simulink model "Model2_V032_R_T4"  (R2023a)
settings: Solver=ode14x  StartTime=0.0  StopTime=Inf  FixedStep=ts  MaxStep=ts  RelTol=1e-5
values from neighbouring files (symbols this model uses):
  ausrollen_a_v = parameters.ausrollen_a_v    [efficiencycalc.m]    (also in parameters_initials.mat = 1)
  bremspunkte = parameters.bremspunkte    [efficiencycalc.m]    (also in parameters_initials.mat = [6100  280  8; 10400  500  3; 14100  550  8; 17729  0  1])
  brennstoffzellen_eta_kennfeld = parameters.brennstoffzellen_eta_kennfeld    [efficiencycalc.m]    (also in parameters_initials.mat = )
  brennstoffzellen_ui_kennfeld = parameters.brennstoffzellen_ui_kennfeld    [efficiencycalc.m]    (also in parameters_initials.mat = )
  coeffs_motor_moment = parameters.coeffs_motor_moment    [efficiencycalc.m]    (also in parameters_initials.mat = [30 30 30 5 7.5 10 0 0 0 6000 6000 6000 ... (30 elements, 3x)
  coeffs_motor_wirkungsgrad = parameters.coeffs_motor_wirkungsgrad    [efficiencycalc.m]    (also in parameters_initials.mat = [30 30 30 5 7.5 10 0 0 0 6000 6000 6000 ... (39 elements, 3x)
  fahrzeug_parameter = parameters.fahrzeug_parameter    [efficiencycalc.m]    (also in parameters_initials.mat = )
  strategie_parameter = parameters.strategie_parameter    [efficiencycalc.m]    (also in parameters_initials.mat = )
  strecke = parameters.strecke    [efficiencycalc.m]    (also in parameters_initials.mat = )
  ts = parameters.ts    [efficiencycalc.m]    (also in parameters_initials.mat = 0.01)
  U_moment = parameters.U_moment    [efficiencycalc.m]    (also in parameters_initials.mat = [30 3])
  U_wirkungsgrad = parameters.U_wirkungsgrad    [efficiencycalc.m]    (also in parameters_initials.mat = [30 3])
  umwelt_parameter = parameters.umwelt_parameter    [efficiencycalc.m]    (also in parameters_initials.mat = )
  zwangsgas = zeros(length(strecke.x),strecke.Rundenzahl)    [Automatisierung_Model_2.m]    (also in efficiencycalc.m; parameters_initials.mat = [0 0 0 0 0 0 0 0 0 0 0 0 ... (2563 elements, 233x11)])
libraries: simulink x1
(part 1 of 3)
settings Model: Creator=Robin Nedella  LastModifiedBy=Fer
settings SolverCC: NumberNewtonIterations=5  AlgebraicLoopSolver=LineSearch
settings DataIOCC: ReturnWorkspaceOutputs=off
settings DebuggingCC: ParameterOverflowMsg=none  UnderSpecifiedDimensionMsg=warning  ArithmeticOperatorsInVariantConditions=warning
settings ModelReferenceCC: EnableRefExpFcnMdlSchedulingChecks=on
settings SFSimCC: SimUseLocalCustomCode=off  CustomCodeUndefinedFunction=UseInterfaceOnly
settings RTWCC: RTWUseLocalCustomCode=off

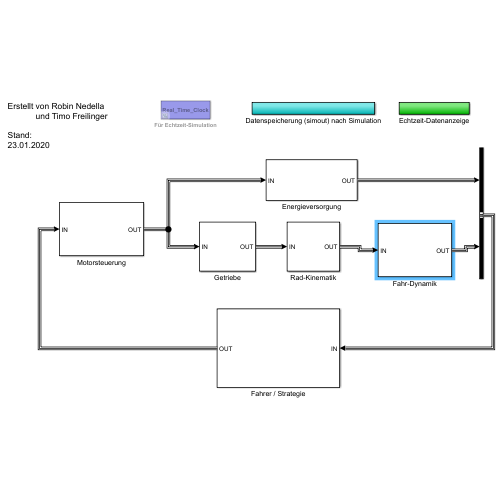
[thumbnail: Simulink's stored preview of the top-level diagram]
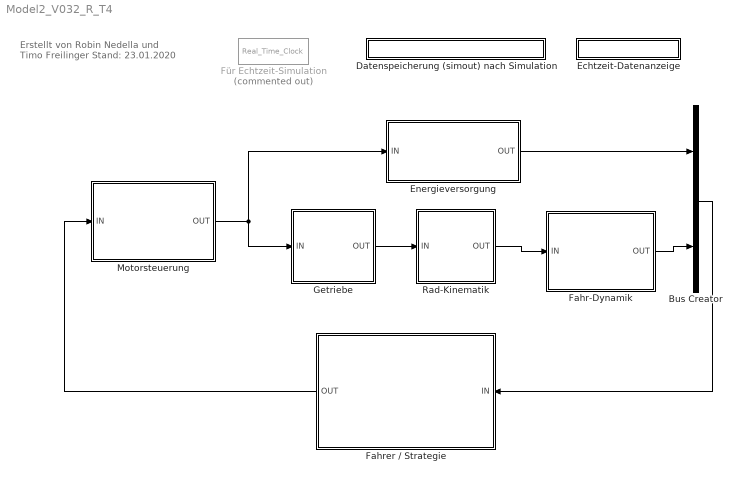
== system Model2_V032_R_T4 ==
  note: Erstellt von Robin Nedella
      | und Timo Freilinger
      |
      | Stand:
      | 23.01.2020
  Bus Creator : BusCreator  Inputs=2
  Datenspeicherung (simout) nach Simulation : Subsystem
  Echtzeit-Datenanzeige : Subsystem
  Energieversorgung : Subsystem
  Fahr-Dynamik : Subsystem
  Fahrer / Strategie : Subsystem
  Für Echtzeit-Simulation : S-Function  Commented=on  FunctionName=Real_Time_Clock  Parameters=ts,0.5  SFunctionDeploymentMode=off  EnableBusSupport=off
  Getriebe : Subsystem
  Motorsteuerung : Subsystem
  Rad-Kinematik : Subsystem
  wires:
  Fahrer / Strategie/1(OUT) -> Motorsteuerung/1(IN)
  Motorsteuerung/1(OUT) -> Energieversorgung/1(IN), Getriebe/1(IN)
  Getriebe/1(OUT) -> Rad-Kinematik/1(IN)
  Rad-Kinematik/1(OUT) -> Fahr-Dynamik/1(IN)
  Fahr-Dynamik/1(OUT) -> Bus Creator/2
  Energieversorgung/1(OUT) -> Bus Creator/1
  Bus Creator/1 -> Fahrer / Strategie/1(IN)

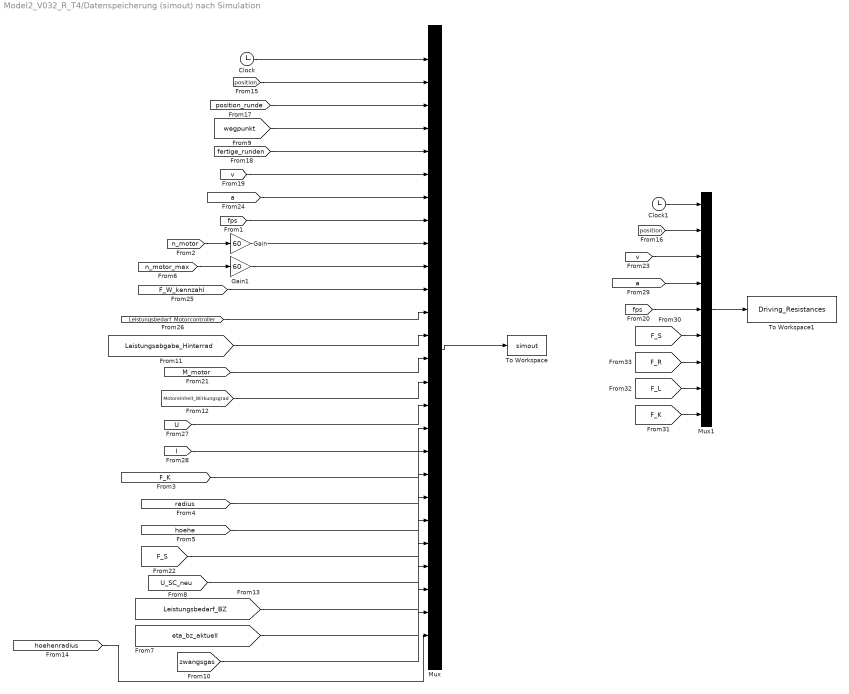
== system Model2_V032_R_T4/Datenspeicherung (simout) nach Simulation ==
  Clock : Clock
  Clock1 : Clock
  Gain : Gain  Gain=60
  Gain1 : Gain  Gain=60
  Mux : Mux  Inputs=26
  Mux1 : Mux  Inputs=9
  To Workspace : ToWorkspace  VariableName=simout  SaveFormat=Timeseries  SampleTime=-1
  To Workspace1 : ToWorkspace  VariableName=Driving_Resistances  SaveFormat=Timeseries  SampleTime=-1
  wires:
  [v] -> Mux/6
  Mux/1 -> To Workspace/1
  [M_motor] -> Mux/14
  Clock/1 -> Mux/1
  [Leistungsabgabe_Hinterrad] -> Mux/13
  [fertige_runden] -> Mux/5
  [a] -> Mux/7
  [n_motor] -> Gain/1
  [F_W_kennzahl] -> Mux/11
  [I] -> Mux/17
  [Leistungsbedarf_Motorcontroller] -> Mux/12
  [position_runde] -> Mux/3
  [U] -> Mux/16
  [position] -> Mux/2
  Gain/1 -> Mux/9
  [F_K] -> Mux/18
  [radius] -> Mux/19
  [hoehe] -> Mux/20
  [F_S] -> Mux/21
  [n_motor_max] -> Gain1/1
  Gain1/1 -> Mux/10
  [U_SC_neu] -> Mux/22
  [Leistungsbedarf_BZ] -> Mux/23
  [eta_bz_aktuell] -> Mux/24
  [wegpunkt] -> Mux/4
  [fps] -> Mux/8
  [zwangsgas] -> Mux/25
  [Motoreinheit_Wirkungsgrad] -> Mux/15
  [hoehenradius] -> Mux/26
  [F_R] -> Mux1/7
  [F_K] -> Mux1/9
  [F_S] -> Mux1/6
  [F_L] -> Mux1/8
  Mux1/1 -> To Workspace1/1
  [position] -> Mux1/2
  Clock1/1 -> Mux1/1
  [v] -> Mux1/3
  [a] -> Mux1/4
  [fps] -> Mux1/5

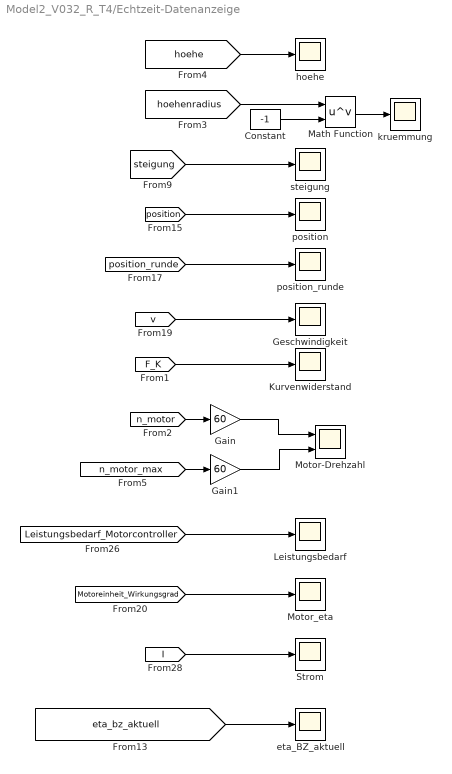
== system Model2_V032_R_T4/Echtzeit-Datenanzeige ==
  Constant : Constant  Value=-1
  Gain : Gain  Gain=60
  Gain1 : Gain  Gain=60
  Geschwindigkeit : Scope
  Kurvenwiderstand : Scope
  Leistungsbedarf : Scope
  Math Function : Math  Operator=pow  SignedPower=on
  Motor-Drehzahl : Scope  NumInputPorts=2
  Motor_eta : Scope
  Strom : Scope
  eta_BZ_aktuell : Scope
  hoehe : Scope
  kruemmung : Scope
  position : Scope
  position_runde : Scope
  steigung : Scope
  wires:
  [I] -> Strom/1
  [v] -> Geschwindigkeit/1
  [n_motor] -> Gain/1
  [position] -> position/1
  [Leistungsbedarf_Motorcontroller] -> Leistungsbedarf/1
  [Motoreinheit_Wirkungsgrad] -> Motor_eta/1
  Gain/1 -> Motor-Drehzahl/1
  [steigung] -> steigung/1
  [position_runde] -> position_runde/1
  [F_K] -> Kurvenwiderstand/1
  [hoehe] -> hoehe/1
  [hoehenradius] -> Math Function/1
  Math Function/1 -> kruemmung/1
  Constant/1 -> Math Function/2
  [eta_bz_aktuell] -> eta_BZ_aktuell/1
  [n_motor_max] -> Gain1/1
  Gain1/1 -> Motor-Drehzahl/2

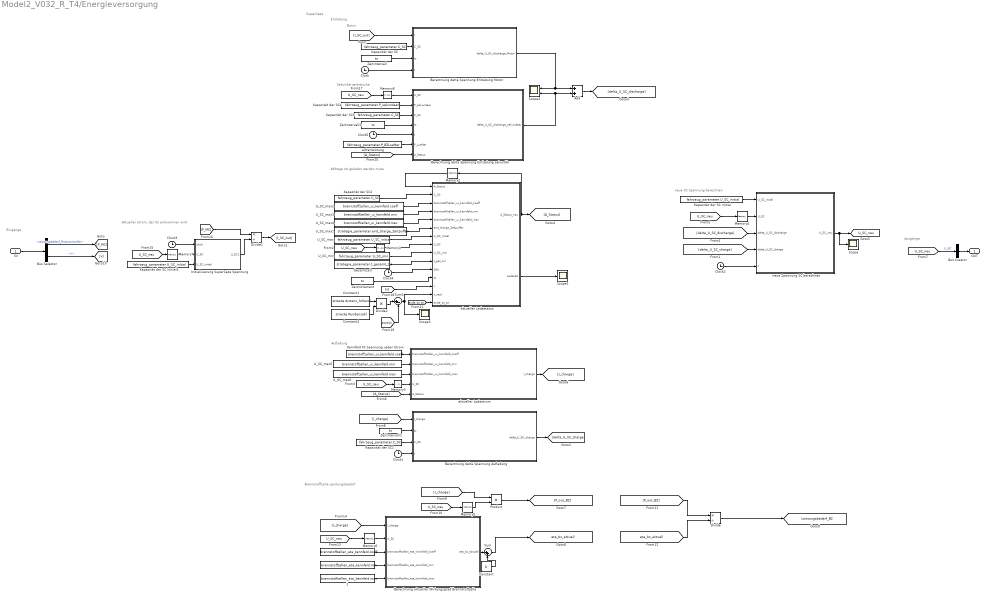
== system Model2_V032_R_T4/Energieversorgung ==
  note: Sekundärverbräuche
  note: Motor
  note: Aktueller Strom, der SC entnommen wird
  note: Brennstoffzelle Leistungsbedarf
  note: Entladung
  note: SuperCaps
  note: Eingänge
  note: Ausgänge
  note: Aufladung
  note: Abfrage ob geladen werden muss
  note: neue SC Spannung berechnen
  IN : Inport
  " " : Constant  Value=brennstoffzellen_eta_kennfeld.min
  "  " : Constant  Value=brennstoffzellen_eta_kennfeld.coeff
  " 1" : Constant  Value=brennstoffzellen_eta_kennfeld.max
  Add : Sum
  Berechnung aktueller Wirkungsgrad Brennstoffzelle : MATLAB Function  TreatAsAtomicUnit=on
  Berechnung delta Spannung Aufladung : MATLAB Function  TreatAsAtomicUnit=on
  Berechnung delta Spannung Entladung Motor : MATLAB Function  TreatAsAtomicUnit=on
  Berechnung delta Spannung Entladung sekundär : MATLAB Function  TreatAsAtomicUnit=on
  Bus Creator : BusCreator  Inputs=1
  Bus Selector : BusSelector  OutputSignals=Leistungsbedarf_Motorcontroller,v
  Clock{,1..5} (6 alike) : Clock
  Constant : Constant  Value=0
  Constant1 : Constant  Value=strecke.distanz_3d(end)
  Constant2 : Constant  Value=strecke.Rundenzahl
  Divide : Product  Inputs=*/
  Divide1 : Product  Inputs=*/
  Divide2 : Product  Inputs=**
  Gesamtzeit : Constant  Value=strategie_parameter.t_gesamt_zul
  Initialisierung SuperCaps Spannung : MATLAB Function  TreatAsAtomicUnit=on
  Kapazität der SC{,1..3} (4 alike) : Constant  Value=fahrzeug_parameter.C_SC
  Kapazität der SC initial : Constant  Value=fahrzeug_parameter.U_SC_initial
  Kapazität der SC initial1 : Constant  Value=fahrzeug_parameter.U_SC_initial
  Kapazität der SC4 : Constant  Value=fahrzeug_parameter.P_sekundaer
  Kennfeld FC Spannung ueber Strom : Constant  Value=brennstoffzellen_ui_kennfeld.coeff
  Lüfterleistung : Constant  Value=fahrzeug_parameter.P_BZLuefter
  Memory{1..8} (8 alike) : Memory
  Product : Product
  Scope : Scope
  Scope1 : Scope
  Scope2 : Scope  NumInputPorts=2
  Scope3 : Scope
  Sum : Sum  Inputs=|++
  Sum1 : Sum  Inputs=|+-
  U_SC_max : Constant  Value=fahrzeug_parameter.U_SC_initial
  U_SC_max1 : Constant  Value=strategie_parameter.end_charge_Zeitpuffer
  U_SC_max2 : Constant  Value=brennstoffzellen_ui_kennfeld.coeff
  U_SC_max3 : Constant  Value=brennstoffzellen_ui_kennfeld.min
  U_SC_max4 : Constant  Value=brennstoffzellen_ui_kennfeld.max
  U_SC_max5 : Constant  Value=brennstoffzellen_ui_kennfeld.min
  U_SC_max6 : Constant  Value=brennstoffzellen_ui_kennfeld.max
  U_SC_min : Constant  Value=fahrzeug_parameter.U_SC_min
  Zeitinkrement : Constant  Value=ts
  Zeitintervall : Constant  Value=ts
  Zeitintervall1 : Constant  Value=ts
  Zeitintervall2 : Constant  Value=ts
  aktueller Ladestatus : MATLAB Function  TreatAsAtomicUnit=on
  aktueller Ladestrom : MATLAB Function  TreatAsAtomicUnit=on
  neue Spannung SC berechnen : MATLAB Function  TreatAsAtomicUnit=on
  OUT : Outport  VectorParamsAs1DForOutWhenUnconnected=off
  tag scope: Leistungsbedarf_BZ=global, U_SC_neu=global, eta_bz_aktuell=global
  wires:
  IN/1 -> Bus Selector/1
  Bus Creator/1 -> OUT/1
  Bus Selector/1 -> [P_MC]  "<Leistungsbedarf_Motorcontroller>"
  [I_SC_out] -> Berechnung delta Spannung Entladung Motor/1(I)
  Kapazität der SC/1 -> Berechnung delta Spannung Entladung Motor/2(C_SC)
  Zeitintervall/1 -> Berechnung delta Spannung Entladung Motor/3(ts)
  Clock/1 -> Berechnung delta Spannung Entladung Motor/4(t)
  aktueller Ladestatus/1(A_Status_neu) -> Memory2/1, [A_Status]
  [U_SC_neu] -> Memory1/1
  Memory1/1 -> aktueller Ladestatus/8(U_SC)
  U_SC_max/1 -> aktueller Ladestatus/7(U_SC_initial)
  U_SC_min/1 -> aktueller Ladestatus/9(U_SC_min)
  Memory2/1 -> aktueller Ladestatus/1(A_Status)
  [U_SC_neu] -> Memory3/1
  Kennfeld FC Spannung ueber Strom/1 -> aktueller Ladestrom/1(brennstoffzellen_ui_kennfeld_koeff)
  Memory3/1 -> aktueller Ladestrom/4(U_SC)
  aktueller Ladestrom/1(I_charge) -> [I_charge]
  [A_Status] -> aktueller Ladestrom/5(A_Status)
  Kapazität der SC1/1 -> Berechnung delta Spannung Aufladung/3(C_SC)
  Zeitintervall1/1 -> Berechnung delta Spannung Aufladung/2(ts)
  Berechnung delta Spannung Aufladung/1(delta_U_SC_charge) -> [delta_U_SC_charge]
  [U_SC_neu] -> Memory4/1
  [delta_U_SC_charge] -> neue Spannung SC berechnen/4(delta_U_SC_charge)
  [delta_U_SC_discharge] -> neue Spannung SC berechnen/3(delta_U_SC_discharge)
  Memory4/1 -> neue Spannung SC berechnen/2(U_SC)
  [U_SC_neu] -> Bus Creator/1  "U_SC"
  Clock1/1 -> Berechnung delta Spannung Aufladung/4(t)
  neue Spannung SC berechnen/1(U_SC_neu) -> Scope/1, [U_SC_neu]
  Clock2/1 -> neue Spannung SC berechnen/5(t)
  Kapazität der SC initial/1 -> neue Spannung SC berechnen/1(U_SC_initial)
  [I_charge] -> Berechnung delta Spannung Aufladung/1(I_charge)
  [U_SC_neu] -> Memory5/1
  Product/1 -> [P_out_BZ]
  [I_charge] -> Product/1
  Memory5/1 -> Product/2
  "  "/1 -> Berechnung aktueller Wirkungsgrad Brennstoffzelle/3(brennstoffzellen_eta_kennfeld_koeff)
  " "/1 -> Berechnung aktueller Wirkungsgrad Brennstoffzelle/4(brennstoffzellen_eta_kennfeld_min)
  Berechnung aktueller Wirkungsgrad Brennstoffzelle/1(eta_bz_aktuell) -> Sum/1
  [P_out_BZ] -> Divide/1
  [eta_bz_aktuell] -> Divide/2
  Divide/1 -> [Leistungsbedarf_BZ]
  " 1"/1 -> Berechnung aktueller Wirkungsgrad Brennstoffzelle/5(brennstoffzellen_eta_kennfeld_max)
  [I_charge] -> Berechnung aktueller Wirkungsgrad Brennstoffzelle/1(I_charge)
  [U_SC_neu] -> Memory6/1
  Memory6/1 -> Berechnung aktueller Wirkungsgrad Brennstoffzelle/2(U_SC)
  [U_SC_neu] -> Memory7/1
  [P_MC] -> Divide1/1
  Divide1/1 -> [I_SC_out]
  Memory7/1 -> Initialisierung SuperCaps Spannung/2(U_SC)
  Clock3/1 -> Initialisierung SuperCaps Spannung/1(clock)
  Kapazität der SC initial1/1 -> Initialisierung SuperCaps Spannung/3(U_SC_initial)
  Initialisierung SuperCaps Spannung/1(U_SC1) -> Divide1/2
  Gesamtzeit/1 -> aktueller Ladestatus/10(t_ges_zul)
  Clock4/1 -> aktueller Ladestatus/11(Zeit)
  Kapazität der SC2/1 -> aktueller Ladestatus/2(C_SC)
  U_SC_max1/1 -> aktueller Ladestatus/6(end_charge_Zeitpuffer)
  Zeitinkrement/1 -> aktueller Ladestatus/12(ts)
  U_SC_max2/1 -> aktueller Ladestatus/3(brennstoffzellen_ui_kennfeld_koeff)
  U_SC_max3/1 -> aktueller Ladestatus/4(brennstoffzellen_ui_kennfeld_min)
  U_SC_max4/1 -> aktueller Ladestatus/5(brennstoffzellen_ui_kennfeld_max)
  aktueller Ladestatus/2(Ladezeit) -> Scope1/1
  U_SC_max5/1 -> aktueller Ladestrom/2(brennstoffzellen_ui_kennfeld_min)
  U_SC_max6/1 -> aktueller Ladestrom/3(brennstoffzellen_ui_kennfeld_max)
  Add/1 -> [delta_U_SC_discharge]
  Berechnung delta Spannung Entladung Motor/1(delta_U_SC_discharge_Motor) -> Scope2/1, Add/1
  Kapazität der SC3/1 -> Berechnung delta Spannung Entladung sekundär/3(C_SC)
  Zeitintervall2/1 -> Berechnung delta Spannung Entladung sekundär/4(ts)
  Clock5/1 -> Berechnung delta Spannung Entladung sekundär/5(t)
  [U_SC_neu] -> Memory8/1
  Memory8/1 -> Berechnung delta Spannung Entladung sekundär/1(U_SC)
  Kapazität der SC4/1 -> Berechnung delta Spannung Entladung sekundär/2(P_sekundaer)
  Berechnung delta Spannung Entladung sekundär/1(delta_U_SC_discharge_sekundaer) -> Add/2, Scope2/2
  Sum/1 -> [eta_bz_aktuell]
  Constant/1 -> Sum/2
  Bus Selector/2 -> [v]  "<v>"
  [v] -> aktueller Ladestatus/13(v)
  Sum1/1 -> Scope3/1, aktueller Ladestatus/14(x_rest)
  [position] -> Sum1/2
  Divide2/1 -> Sum1/1
  Constant1/1 -> Divide2/1
  Constant2/1 -> Divide2/2
  Lüfterleistung/1 -> Berechnung delta Spannung Entladung sekundär/6(P_Luefter)
  [A_Status] -> Berechnung delta Spannung Entladung sekundär/7(A_Status)
  [ende_bz_an] -> aktueller Ladestatus/15(ende_bz_an)

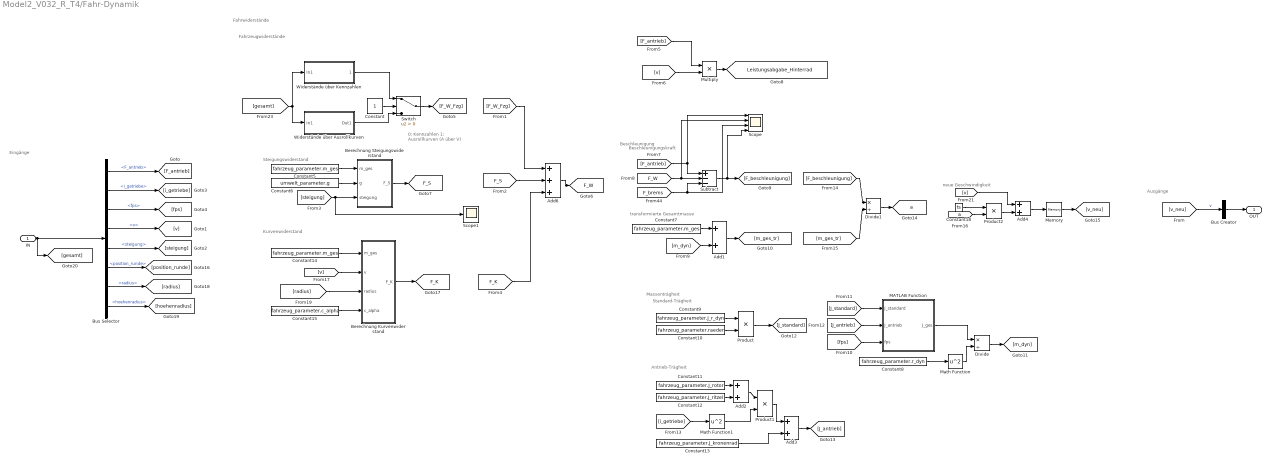
== system Model2_V032_R_T4/Fahr-Dynamik ==
  note: 0: Kennzahlen
      | 1: Ausrollkurven (A über V)
  note: Beschleunigung
  note: Antrieb-Trägheit
  note: Massenträgheit
  note: Standard-Trägheit
  note: Beschleunigungskraft
  note: neue Geschwindigkeit
  note: Ausgänge
  note: Eingänge
  note: transformierte Gesamtmasse
  note: Fahrwiderstände
  note: Fahrzeugwiderstände
  note: Kurvenwiderstand
  note: Steigungswiderstand
  IN : Inport
  Add{1..4} (4 alike) : Sum
  Add6 : Sum  Inputs=+++
  Berechnung Kurvenwiderstand : MATLAB Function  TreatAsAtomicUnit=on
  Berechnung Steigungswiderstand : MATLAB Function  TreatAsAtomicUnit=on
  Bus Creator : BusCreator  Inputs=1
  Bus Selector : BusSelector  OutputSignals=F_antrieb,i_getriebe,fps,v,steigung,position_runde,radius,hoehenradius
  Constant : Constant
  Constant10 : Constant  Value=fahrzeug_parameter.raeder
  Constant11 : Constant  Value=fahrzeug_parameter.J_rotor
  Constant12 : Constant  Value=fahrzeug_parameter.J_ritzel
  Constant13 : Constant  Value=fahrzeug_parameter.J_kronenrad
  Constant14 : Constant  Value=fahrzeug_parameter.m_ges
  Constant15 : Constant  Value=fahrzeug_parameter.c_alpha
  Constant18 : Constant  Value=ts
  Constant5 : Constant  Value=fahrzeug_parameter.m_ges
  Constant6 : Constant  Value=umwelt_parameter.g
  Constant7 : Constant  Value=fahrzeug_parameter.m_ges
  Constant8 : Constant  Value=fahrzeug_parameter.r_dyn
  Constant9 : Constant  Value=fahrzeug_parameter.J_r_dyn
  Divide : Product  Inputs=*/
  Divide1 : Product  Inputs=*/
  MATLAB Function : MATLAB Function  TreatAsAtomicUnit=on
  Math Function : Math  Operator=square  SignedPower=on
  Math Function1 : Math  Operator=square  SignedPower=on
  Memory : Memory
  Multiply : Product
  Product : Product
  Product1 : Product
  Product2 : Product
  Scope : Scope  NumInputPorts=4
  Scope1 : Scope
  Subtract : Sum  Inputs=+--
  Switch : Switch  Criteria=u2 > Threshold  SaturateOnIntegerOverflow=off  InputSameDT=off
  Widerstände über Ausrollkurven : Subsystem
  Widerstände über Kennzahlen : Subsystem
  OUT : Outport  VectorParamsAs1DForOutWhenUnconnected=off
  tag scope: F_K=global, F_S=global, F_W=global, Leistungsabgabe_Hinterrad=global, a=global
  wires:
  [v_neu] -> Bus Creator/1  "v"
  [J_antrieb] -> MATLAB Function/2(J_antrieb)
  Divide/1 -> [m_dyn]
  MATLAB Function/1(J_ges) -> Divide/1
  [F_antrieb] -> Subtract/1, Scope/1
  Constant11/1 -> Add2/1
  [F_W] -> Scope/2, Subtract/2
  Add3/1 -> [J_antrieb]
  Constant9/1 -> Product/1
  Constant8/1 -> Math Function/1
  Bus Selector/3 -> [fps]  "<fps>"
  [m_dyn] -> Add1/2
  Product/1 -> [J_standard]
  Constant13/1 -> Add3/2
  [m_ges_tr] -> Divide1/2
  Bus Selector/1 -> [F_antrieb]  "<F_antrieb>"
  [i_getriebe] -> Math Function1/1
  [a] -> Product2/2
  Math Function/1 -> Divide/2
  Divide1/1 -> [a]
  [F_beschleunigung] -> Divide1/1
  Constant7/1 -> Add1/1
  Bus Selector/2 -> [i_getriebe]  "<i_getriebe>"
  Math Function1/1 -> Product1/2
  Subtract/1 -> Scope/4, [F_beschleunigung]
  Bus Creator/1 -> OUT/1
  Constant12/1 -> Add2/2
  [J_standard] -> MATLAB Function/1(J_standard)
  IN/1 -> [gesamt], Bus Selector/1
  Add2/1 -> Product1/1
  Constant10/1 -> Product/2
  [fps] -> MATLAB Function/3(fps)
  Bus Selector/5 -> [steigung]  "<steigung>"
  Add1/1 -> [m_ges_tr]
  Product1/1 -> Add3/1
  Bus Selector/4 -> [v]  "<v>"
  Bus Selector/6 -> [position_runde]  "<position_runde>"
  Constant18/1 -> Product2/1
  Product2/1 -> Add4/2
  [v] -> Add4/1
  Add4/1 -> Memory/1
  Memory/1 -> [v_neu]
  Bus Selector/7 -> [radius]  "<radius>"
  Bus Selector/8 -> [hoehenradius]  "<hoehenradius>"
  [gesamt] -> Widerstände über Kennzahlen/1(In1), Widerstände über Ausrollkurven/1(In1)
  Switch/1 -> [F_W_Fzg]
  Widerstände über Ausrollkurven/1(Out1) -> Switch/3
  Constant15/1 -> Berechnung Kurvenwiderstand/4(c_alpha)
  Berechnung Kurvenwiderstand/1(F_K) -> [F_K]
  Berechnung Steigungswiderstand/1(F_S) -> [F_S]
  Constant5/1 -> Berechnung Steigungswiderstand/1(m_ges)
  Constant6/1 -> Berechnung Steigungswiderstand/2(g)
  [v] -> Berechnung Kurvenwiderstand/2(v)
  Constant14/1 -> Berechnung Kurvenwiderstand/1(m_ges)
  [radius] -> Berechnung Kurvenwiderstand/3(radius)
  Add6/1 -> [F_W]
  [F_W_Fzg] -> Add6/1
  [F_S] -> Add6/2
  Constant/1 -> Switch/2
  [F_K] -> Add6/3
  [F_brems] -> Scope/3, Subtract/3
  [v] -> Multiply/2
  [F_antrieb] -> Multiply/1
  Multiply/1 -> [Leistungsabgabe_Hinterrad]
  [steigung] -> Scope1/1, Berechnung Steigungswiderstand/3(steigung)
  Widerstände über Kennzahlen/1(1) -> Switch/1

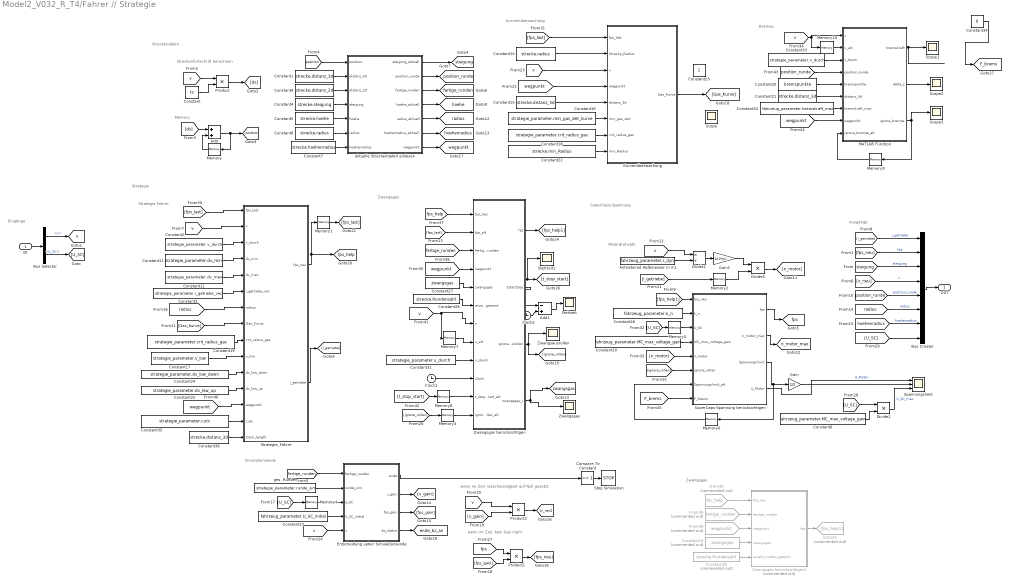
== system Model2_V032_R_T4/Fahrer // Strategie ==
  note: Kurvenüberwachung
  note: Strategie
  note: Simulationsende
  note: Streckendaten
  note: Streckenfortschritt berechnen
  note: Ausgänge
  note: Eingänge
  note: Motordrehzahl
  note: Strategie Fahrer
  note: wenn im Ziel: kein Gas mehr
  note: wenn im Ziel: Geschwindigkeit auf Null gesetzt
  note: SuperCaps-Spannung
  note: Zwangsgas
  note: Zwangsgas
  note: Bremse
  note: Memory
  IN : Inport
  Add : Sum
  Add1 : Sum  Inputs=-+
  Antriebsrad Halbmesser in m1 : Constant  Value=fahrzeug_parameter.r_dyn
  Bus Creator : BusCreator  Inputs=8
  Bus Selector : BusSelector  OutputSignals=signal2.v,signal1.U_SC
  Clock1 : Clock
  Clock2 : Clock
  Compare To Constant : simulink/Logic and Bit Operations/Compare To Constant  relop===  const=1  OutDataTypeStr=boolean
  Constant : Constant  Value=ts
  Constant{1,15,21,36} (4 alike) : Constant  Value=strecke.distanz_3d
  Constant10 : Constant  Value=fahrzeug_parameter.MC_max_voltage_gain
  Constant11 : Constant  Value=strategie_parameter.dv_min
  Constant12 : Constant  Value=strategie_parameter.dv_max
  Constant13 : Constant  Value=fahrzeug_parameter.U_SC_initial
  Constant14 : Constant  Value=strecke.radius
  Constant16 : Constant  Value=strategie_parameter.min_gas_zeit_kurve
  Constant17 : Constant  Value=strategie_parameter.v_low
  Constant18 : Constant  Value=strategie_parameter.crit_radius_gas
  Constant19 : Constant  Value=strategie_parameter.crit_radius_gas
  Constant2 : Constant  Value=strategie_parameter.v_durch
  Constant20 : Constant  Value=bremspunkte
  Constant22 : Constant  Value=strecke.min_Radius
  Constant23 : Constant
  Constant24 : Constant  Value=strategie_parameter.dv_low_down
  Constant25 : Constant  Value=strategie_parameter.dv_low_up
  Constant26 : Constant  Value=fahrzeug_parameter.k_n
  Constant27 : Constant  Value=zwangsgas
  Constant28 : Constant  Value=strecke.Rundenzahl
  Constant29 : Constant  Commented=on  Value=zwangsgas
  Constant3 : Constant  Value=strategie_parameter.i_getriebe_vec
  Constant30 : Constant  Commented=on  Value=strecke.Rundenzahl
  Constant31 : Constant  Value=strategie_parameter.v_durch
  Constant32 : Constant  Value=fahrzeug_parameter.bremskraft_max  VectorParams1D=off
  Constant33 : Constant  Value=strategie_parameter.v_durch
  Constant34 : Constant  Value=0
  Constant35 : Constant  Value=strategie_parameter.cuts
  Constant4 : Constant  Value=strecke.steigung
  Constant5 : Constant  Value=strecke.hoehe
  Constant6 : Constant  Value=fahrzeug_parameter.MC_max_voltage_gain
  Constant7 : Constant  Value=strecke.hoehenradius
  Constant8 : Constant  Value=strecke.radius
  Constant9 : Constant  Value=strecke.distanz_2d
  Divide1 : Product  Inputs=*/
  Divide2 : Product  Inputs=**
  Divide5 : Product  Inputs=**
  Entscheidung ueber Simulationsende : MATLAB Function  TreatAsAtomicUnit=on
  From38 : From  Commented=on  GotoTag=wegpunkt  TagVisibility=global
  From39 : From  Commented=on  GotoTag=fertige_runden  TagVisibility=global
  From40 : From  Commented=on  GotoTag=fps_help  TagVisibility=global
  Gain : Gain  Gain=10
  Gain1 : Gain  Gain=1/(2*pi)
  Goto25 : Goto  Commented=on  GotoTag=fps_help1
  Kurvenüberwachung : MATLAB Function  TreatAsAtomicUnit=on
  MATLAB Function : MATLAB Function  TreatAsAtomicUnit=on
  Memory{,1..10} (11 alike) : Memory
  Product : Product
  Product1 : Product
  Product2 : Product
  Scope{,1..3} (4 alike) : Scope
  Spannungslimit : Scope  NumInputPorts=3
  Stehzeit : Scope
  Stehzeit1 : Scope
  Stop Simulation : Stop
  Strategie_Fahrer : MATLAB Function  TreatAsAtomicUnit=on
  SuperCaps-Spannung berücksichtigen : MATLAB Function  TreatAsAtomicUnit=on
  Zwangsausrollen : Scope
  Zwangsgas : Scope
  Zwangsgas berücksichtigen : MATLAB Function  TreatAsAtomicUnit=on
  Zwangsgas berücksichtigen1 : MATLAB Function  Commented=on  TreatAsAtomicUnit=on
  aktuelle Streckendaten einlesen : MATLAB Function  TreatAsAtomicUnit=on
  ges. Runden : Constant  Value=strategie_parameter.runde_sim
  OUT : Outport  VectorParamsAs1DForOutWhenUnconnected=off
  tag scope: F_brems=global, ende_bz_an=global, fertige_runden=global, fps=global, fps_help=global, hoehe=global, hoehenradius=global, n_motor_max=global, position=global, position_runde=global, radius=global, steigung=global, v=global, wegpunkt=global, zwangsgas=global
  wires:
  IN/1 -> Bus Selector/1
  [steigung] -> Bus Creator/3  "steigung"
  [v] -> Product/1
  Constant/1 -> Product/2
  Product/1 -> [ds]
  [ds] -> Add/1
  Add/1 -> Memory/1, [position]
  Memory/1 -> Add/2
  Constant1/1 -> aktuelle Streckendaten einlesen/2(distanz_3d)
  [position] -> aktuelle Streckendaten einlesen/1(position)
  aktuelle Streckendaten einlesen/1(steigung_aktuell) -> [steigung]
  aktuelle Streckendaten einlesen/2(position_runde) -> [position_runde]
  aktuelle Streckendaten einlesen/3(fertige_runden) -> [fertige_runden]
  [fertige_runden] -> Entscheidung ueber Simulationsende/1(fertige_runden)
  ges. Runden/1 -> Entscheidung ueber Simulationsende/2(runde_sim)
  Entscheidung ueber Simulationsende/1(ende) -> Compare To Constant/1
  Compare To Constant/1 -> Stop Simulation/1
  [v] -> Strategie_Fahrer/2(v)
  Constant2/1 -> Strategie_Fahrer/3(v_durch)
  [i_getriebe] -> Bus Creator/1  "i_getriebe"
  Constant3/1 -> Strategie_Fahrer/6(i_getriebe_vec)
  Strategie_Fahrer/2(i_getriebe) -> [i_getriebe]
  [fps_neu] -> Bus Creator/2  "fps"
  Bus Creator/1 -> OUT/1
  [v_neu] -> Bus Creator/4  "v"
  Bus Selector/1 -> [v]  "<v>"
  [position_runde] -> Bus Creator/5  "position_runde"
  Constant4/1 -> aktuelle Streckendaten einlesen/4(steigung)
  Constant5/1 -> aktuelle Streckendaten einlesen/5(hoehe)
  aktuelle Streckendaten einlesen/4(hoehe_aktuell) -> [hoehe]
  Gain1/1 -> Divide5/1
  [v] -> Divide1/1
  Antriebsrad Halbmesser in m1/1 -> Divide1/2
  [i_getriebe] -> Memory2/1
  Divide1/1 -> Gain1/1
  Divide5/1 -> [n_motor]
  Memory2/1 -> Divide5/2
  Constant8/1 -> aktuelle Streckendaten einlesen/6(radius)
  aktuelle Streckendaten einlesen/5(radius_aktuell) -> [radius]
  [radius] -> Bus Creator/6  "radius"
  Bus Selector/2 -> [U_SC]  "<U_SC>"
  Constant7/1 -> aktuelle Streckendaten einlesen/7(hoehenradius)
  aktuelle Streckendaten einlesen/6(hoehenradius_aktuell) -> [hoehenradius]
  [hoehenradius] -> Bus Creator/7  "hoehenradius"
  Constant9/1 -> aktuelle Streckendaten einlesen/3(distanz_2d)
  [radius] -> Strategie_Fahrer/7(radius)
  Constant10/1 -> SuperCaps-Spannung berücksichtigen/4(MC_max_voltage_gain)
  Constant11/1 -> Strategie_Fahrer/4(dv_min)
  Constant12/1 -> Strategie_Fahrer/5(dv_max)
  Entscheidung ueber Simulationsende/2(v_gain) -> [v_gain]
  Entscheidung ueber Simulationsende/3(fps_gain) -> [fps_gain]
  [U_SC] -> Memory4/1
  Memory4/1 -> Entscheidung ueber Simulationsende/3(U_SC)
  Constant13/1 -> Entscheidung ueber Simulationsende/4(U_SC_initial)
  Strategie_Fahrer/1(fps_neu) -> [fps_help], Memory1/1
  Product2/1 -> [v_neu]
  [v] -> Product2/1
  [v_gain] -> Product2/2
  Constant14/1 -> Kurvenüberwachung/2(Strecke_Radius)
  aktuelle Streckendaten einlesen/7(wegpunkt) -> [wegpunkt]
  [wegpunkt] -> Kurvenüberwachung/4(wegpunkt)
  Constant15/1 -> Kurvenüberwachung/5(distanz_3d)
  [v] -> Kurvenüberwachung/3(v)
  Constant16/1 -> Kurvenüberwachung/6(min_gas_zeit)
  Kurvenüberwachung/1(Gas_Kurve) -> [Gas_Kurve]
  [Gas_Kurve] -> Strategie_Fahrer/8(Gas_Kurve)
  Constant17/1 -> Strategie_Fahrer/10(v_low)
  [v] -> Entscheidung ueber Simulationsende/5(v)
  Constant18/1 -> Kurvenüberwachung/7(crit_radius_gas)
  Constant19/1 -> Strategie_Fahrer/9(crit_radius_gas)
  SuperCaps-Spannung berücksichtigen/1(fps) -> [fps]
  [fps] -> Product1/1
  [fps_gain] -> Product1/2
  Product1/1 -> [fps_neu]
  Constant24/1 -> Strategie_Fahrer/11(dv_low_down)
  Constant25/1 -> Strategie_Fahrer/12(dv_low_up)
  [U_SC] -> Bus Creator/8
  Memory1/1 -> [fps_last]
  [fps_last] -> Strategie_Fahrer/1(fps_last)
  [fps_last] -> Kurvenüberwachung/1(fps_last)
  Constant22/1 -> Kurvenüberwachung/8(min_Radius)
  Constant26/1 -> SuperCaps-Spannung berücksichtigen/2(k_n)
  [U_SC] -> Memory5/1
  Memory5/1 -> SuperCaps-Spannung berücksichtigen/3(U_SC)
  [n_motor] -> SuperCaps-Spannung berücksichtigen/5(n_motor)
  SuperCaps-Spannung berücksichtigen/2(n_motor_max) -> [n_motor_max]
  [fps_help1] -> SuperCaps-Spannung berücksichtigen/1(fps_neu)
  Zwangsgas berücksichtigen/1(fps) -> [fps_help1]
  [fertige_runden] -> Zwangsgas berücksichtigen/3(fertige_runden)
  Constant28/1 -> Zwangsgas berücksichtigen/6(anzahl_runden_gesamt)
  [fps_help] -> Zwangsgas berücksichtigen/1(fps_neu)
  [wegpunkt] -> Zwangsgas berücksichtigen/4(wegpunkt)
  Constant27/1 -> Zwangsgas berücksichtigen/5(zwangsgas)
  From40/1 -> Zwangsgas berücksichtigen1/1(fps_neu)
  From38/1 -> Zwangsgas berücksichtigen1/3(wegpunkt)
  Constant30/1 -> Zwangsgas berücksichtigen1/5(anzahl_runden_gesamt)
  Zwangsgas berücksichtigen1/1(fps) -> Goto25/1
  Constant29/1 -> Zwangsgas berücksichtigen1/4(zwangsgas)
  From39/1 -> Zwangsgas berücksichtigen1/2(fertige_runden)
  Zwangsgas berücksichtigen/2(tstartstop) -> Stehzeit1/1, [t_stop_start], Add1/1
  [v] -> Zwangsgas berücksichtigen/7(v), Memory7/1
  Memory7/1 -> Zwangsgas berücksichtigen/8(v_alt)
  Constant31/1 -> Zwangsgas berücksichtigen/9(v_durch)
  Clock1/1 -> Zwangsgas berücksichtigen/10(clock)
  [t_stop_start] -> Memory8/1
  Memory8/1 -> Zwangsgas berücksichtigen/11(t_stop_start_alt)
  Clock2/1 -> Add1/2
  Add1/1 -> Stehzeit/1
  [fps_last] -> Zwangsgas berücksichtigen/2(fps_alt)
  Zwangsgas berücksichtigen/3(ignore_zwangsausrollen) -> [ignore_rollen], Zwangsausrollen/1
  [ignore_rollen] -> SuperCaps-Spannung berücksichtigen/6(ignore_rollen)
  Zwangsgas berücksichtigen/4(zwangsgas_i) -> Zwangsgas/1, [zwangsgas]
  [ignore_rollen] -> Memory3/1
  Memory3/1 -> Zwangsgas berücksichtigen/12(ignore_zwangsausrollen_alt)
  SuperCaps-Spannung berücksichtigen/3(Spannungslimit) -> Gain/1, Memory6/1
  Memory6/1 -> SuperCaps-Spannung berücksichtigen/7(Spannungslimit_alt)
  [U_SC] -> Divide2/1
  SuperCaps-Spannung berücksichtigen/4(U_Motor) -> Spannungslimit/1  "U_Motor"
  Divide2/1 -> Spannungslimit/3  "U_SC_max"
  Constant6/1 -> Divide2/2
  Gain/1 -> Spannungslimit/2
  [v] -> Memory10/1, MATLAB Function/1(v)
  [position_runde] -> MATLAB Function/4(position_runde)
  Constant20/1 -> MATLAB Function/5(bremspunkte)
  MATLAB Function/1(bremskraft) -> Scope1/1
  Constant21/1 -> MATLAB Function/6(distanz_3d)
  [wegpunkt] -> MATLAB Function/8(wegpunkt)
  Constant32/1 -> MATLAB Function/7(bremskraft_max)
  [F_brems] -> SuperCaps-Spannung berücksichtigen/8(F_brems)
  MATLAB Function/2(delta_s) -> Scope2/1
  MATLAB Function/3(ignore_bremse) -> Memory9/1, Scope3/1
  Memory9/1 -> MATLAB Function/9(ignore_bremse_alt)
  Constant33/1 -> MATLAB Function/3(v_durch)
  Memory10/1 -> MATLAB Function/2(v_alt)
  Entscheidung ueber Simulationsende/4(bz_status) -> [ende_bz_an]
  Constant34/1 -> [F_brems]
  [wegpunkt] -> Strategie_Fahrer/13(wegpunkt)
  Constant35/1 -> Strategie_Fahrer/14(cuts)
  Constant36/1 -> Strategie_Fahrer/15(track_length)

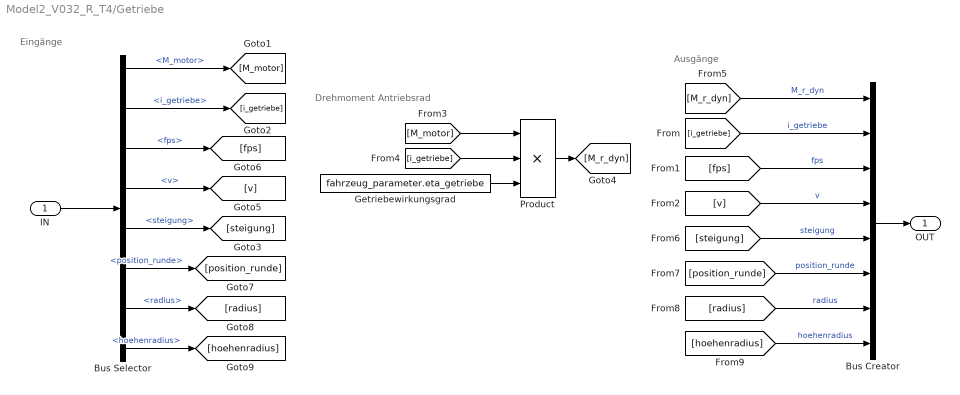
== system Model2_V032_R_T4/Getriebe ==
  note: Drehmoment Antriebsrad
  note: Ausgänge
  note: Eingänge
  IN : Inport
  Bus Creator : BusCreator  Inputs=8
  Bus Selector : BusSelector  OutputSignals=M_motor,i_getriebe,fps,v,steigung,position_runde,radius,hoehenradius
  Getriebewirkungsgrad : Constant  Value=fahrzeug_parameter.eta_getriebe
  Product : Product  Inputs=3
  OUT : Outport  VectorParamsAs1DForOutWhenUnconnected=off
  wires:
  IN/1 -> Bus Selector/1
  [M_motor] -> Product/1
  [i_getriebe] -> Product/2
  [M_r_dyn] -> Bus Creator/1  "M_r_dyn"
  Product/1 -> [M_r_dyn]
  Bus Selector/1 -> [M_motor]  "<M_motor>"
  Bus Selector/3 -> [fps]  "<fps>"
  Bus Selector/5 -> [steigung]  "<steigung>"
  Bus Selector/4 -> [v]  "<v>"
  Bus Selector/2 -> [i_getriebe]  "<i_getriebe>"
  Bus Creator/1 -> OUT/1
  [i_getriebe] -> Bus Creator/2  "i_getriebe"
  [fps] -> Bus Creator/3  "fps"
  [v] -> Bus Creator/4  "v"
  [steigung] -> Bus Creator/5  "steigung"
  Getriebewirkungsgrad/1 -> Product/3
  Bus Selector/6 -> [position_runde]  "<position_runde>"
  [position_runde] -> Bus Creator/6  "position_runde"
  Bus Selector/7 -> [radius]  "<radius>"
  [radius] -> Bus Creator/7  "radius"
  Bus Selector/8 -> [hoehenradius]  "<hoehenradius>"
  [hoehenradius] -> Bus Creator/8  "hoehenradius"

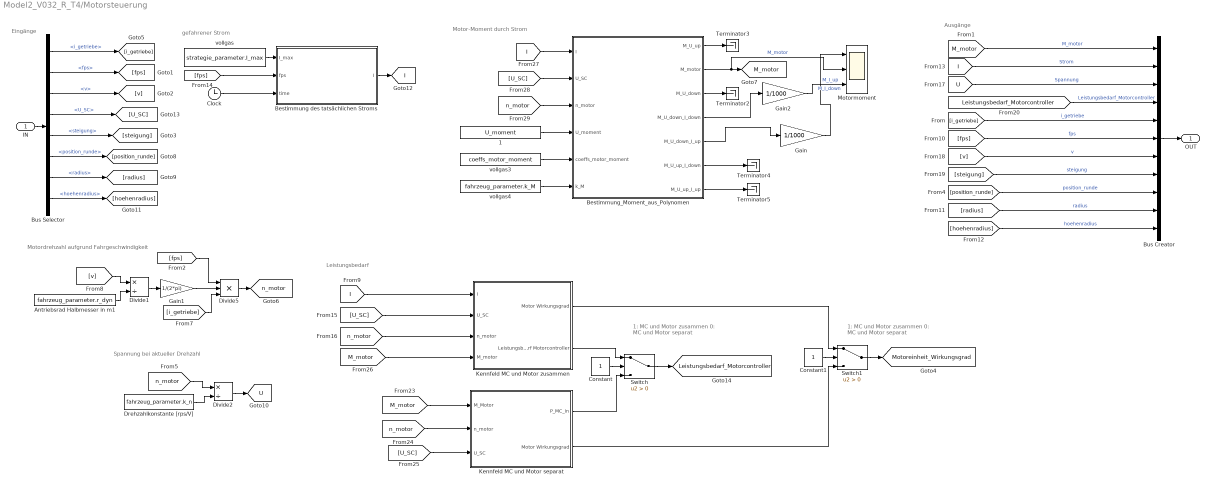
== system Model2_V032_R_T4/Motorsteuerung ==
  note: Leistungsbedarf
  note: gefahrener Strom
  note: Spannung bei aktueller Drehzahl
  note: Motordrehzahl aufgrund Fahrgeschwindigkeit
  note: Ausgänge
  note: Eingänge
  note: 1: MC und Motor zusammen
      | 0: MC und Motor separat
  note: 1: MC und Motor zusammen
      | 0: MC und Motor separat
  note: Motor-Moment durch Strom
  IN : Inport
  " 1" : Constant  Value=U_moment  VectorParams1D=off
  Antriebsrad Halbmesser in m1 : Constant  Value=fahrzeug_parameter.r_dyn
  Bestimmung des tatsächlichen Stroms : MATLAB Function  TreatAsAtomicUnit=on
  Bestimmung_Moment_aus_Polynomen : MATLAB Function  TreatAsAtomicUnit=on
  Bus Creator : BusCreator  Inputs=11
  Bus Selector : BusSelector  OutputSignals=i_getriebe,fps,v,U_SC,steigung,position_runde,radius,hoehenradius
  Clock : Clock
  Constant : Constant
  Constant1 : Constant
  Divide1 : Product  Inputs=*/
  Divide2 : Product  Inputs=*/
  Divide5 : Product  Inputs=***
  "Drehzahlkonstante [rps/V] " : Constant  Value=fahrzeug_parameter.k_n
  Gain : Gain  Gain=1/1000
  Gain1 : Gain  Gain=1/(2*pi)
  Gain2 : Gain  Gain=1/1000
  Kennfeld MC und Motor separat : Subsystem
  Kennfeld MC und Motor zusammen : Subsystem
  Motormoment : Scope  NumInputPorts=3
  Switch : Switch  Criteria=u2 > Threshold  SaturateOnIntegerOverflow=off  InputSameDT=off
  Switch1 : Switch  Criteria=u2 > Threshold  SaturateOnIntegerOverflow=off  InputSameDT=off
  Terminator{2..5} (4 alike) : Terminator
  vollgas : Constant  Value=strategie_parameter.I_max
  vollgas3 : Constant  Value=coeffs_motor_moment  VectorParams1D=off
  vollgas4 : Constant  Value=fahrzeug_parameter.k_M
  OUT : Outport  VectorParamsAs1DForOutWhenUnconnected=off
  tag scope: I=global, Leistungsbedarf_Motorcontroller=global, M_motor=global, Motoreinheit_Wirkungsgrad=global, U=global, n_motor=global
  wires:
  [M_motor] -> Bus Creator/1  "M_motor"
  [i_getriebe] -> Divide5/3
  Divide5/1 -> [n_motor]
  [v] -> Divide1/1
  Antriebsrad Halbmesser in m1/1 -> Divide1/2
  Divide1/1 -> Gain1/1
  Gain1/1 -> Divide5/2
  "Drehzahlkonstante [rps/V] "/1 -> Divide2/2
  [n_motor] -> Divide2/1
  Divide2/1 -> [U]
  vollgas/1 -> Bestimmung des tatsächlichen Stroms/1(I_max)
  Bestimmung des tatsächlichen Stroms/1(I) -> [I]
  [fps] -> Bestimmung des tatsächlichen Stroms/2(fps)
  [fps] -> Divide5/1
  IN/1 -> Bus Selector/1
  Bus Selector/1 -> [i_getriebe]  "<i_getriebe>"
  Bus Selector/2 -> [fps]  "<fps>"
  Bus Selector/3 -> [v]  "<v>"
  [i_getriebe] -> Bus Creator/5  "i_getriebe"
  Bus Creator/1 -> OUT/1
  Bus Selector/5 -> [steigung]  "<steigung>"
  [fps] -> Bus Creator/6  "fps"
  [v] -> Bus Creator/7  "v"
  [steigung] -> Bus Creator/8  "steigung"
  Bus Selector/6 -> [position_runde]  "<position_runde>"
  [position_runde] -> Bus Creator/9  "position_runde"
  Bus Selector/7 -> [radius]  "<radius>"
  [radius] -> Bus Creator/10  "radius"
  [I] -> Bus Creator/2  "Strom"
  [U] -> Bus Creator/3  "Spannung"
  Bus Selector/8 -> [hoehenradius]  "<hoehenradius>"
  [hoehenradius] -> Bus Creator/11  "hoehenradius"
  [Leistungsbedarf_Motorcontroller] -> Bus Creator/4  "Leistungsbedarf_Motorcontroller"
  Bus Selector/4 -> [U_SC]  "<U_SC>"
  Clock/1 -> Bestimmung des tatsächlichen Stroms/3(time)
  Switch/1 -> [Leistungsbedarf_Motorcontroller]
  Kennfeld MC und Motor zusammen/2(Leistungsbedarf Motorcontroller) -> Switch/1
  Constant/1 -> Switch/2
  Kennfeld MC und Motor separat/1(P_MC_in) -> Switch/3
  [I] -> Kennfeld MC und Motor zusammen/1(I)
  [n_motor] -> Kennfeld MC und Motor zusammen/3(n_motor)
  [M_motor] -> Kennfeld MC und Motor separat/1(M_Motor)
  [n_motor] -> Kennfeld MC und Motor separat/2(n_motor)
  Kennfeld MC und Motor separat/2(Motor Wirkungsgrad) -> Switch1/3
  Constant1/1 -> Switch1/2
  Kennfeld MC und Motor zusammen/1(Motor Wirkungsgrad) -> Switch1/1
  Switch1/1 -> [Motoreinheit_Wirkungsgrad]
  [U_SC] -> Kennfeld MC und Motor zusammen/2(U_SC)
  [U_SC] -> Kennfeld MC und Motor separat/3(U_SC)
  [M_motor] -> Kennfeld MC und Motor zusammen/4(M_motor)
  [n_motor] -> Bestimmung_Moment_aus_Polynomen/3(n_motor)
  [U_SC] -> Bestimmung_Moment_aus_Polynomen/2(U_SC)
  [I] -> Bestimmung_Moment_aus_Polynomen/1(I)
  " 1"/1 -> Bestimmung_Moment_aus_Polynomen/4(U_moment)
  vollgas3/1 -> Bestimmung_Moment_aus_Polynomen/5(coeffs_motor_moment)
  Bestimmung_Moment_aus_Polynomen/7(M_U_up_I_up) -> Terminator5/1
  Bestimmung_Moment_aus_Polynomen/1(M_U_up) -> Terminator3/1
  Bestimmung_Moment_aus_Polynomen/4(M_U_down_I_down) -> Gain2/1
  Bestimmung_Moment_aus_Polynomen/3(M_U_down) -> Terminator2/1
  Bestimmung_Moment_aus_Polynomen/5(M_U_down_I_up) -> Gain/1
  Bestimmung_Moment_aus_Polynomen/6(M_U_up_I_down) -> Terminator4/1
  Bestimmung_Moment_aus_Polynomen/2(M_motor) -> Motormoment/2, [M_motor]  "M_motor"
  vollgas4/1 -> Bestimmung_Moment_aus_Polynomen/6(k_M)
  Gain/1 -> Motormoment/1  "M_I_up"
  Gain2/1 -> Motormoment/3  "M_I_down"

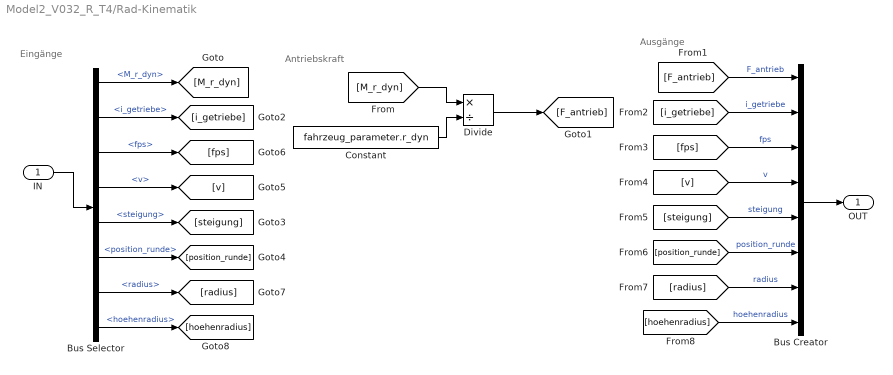
== system Model2_V032_R_T4/Rad-Kinematik ==
  note: Antriebskraft
  note: Ausgänge
  note: Eingänge
  IN : Inport
  Bus Creator : BusCreator  Inputs=8
  Bus Selector : BusSelector  OutputSignals=M_r_dyn,i_getriebe,fps,v,steigung,position_runde,radius,hoehenradius
  Constant : Constant  Value=fahrzeug_parameter.r_dyn
  Divide : Product  Inputs=*/
  OUT : Outport  VectorParamsAs1DForOutWhenUnconnected=off
  wires:
  IN/1 -> Bus Selector/1
  [M_r_dyn] -> Divide/1
  Constant/1 -> Divide/2
  Divide/1 -> [F_antrieb]
  [F_antrieb] -> Bus Creator/1  "F_antrieb"
  Bus Selector/1 -> [M_r_dyn]  "<M_r_dyn>"
  Bus Selector/2 -> [i_getriebe]  "<i_getriebe>"
  Bus Selector/3 -> [fps]  "<fps>"
  Bus Selector/4 -> [v]  "<v>"
  Bus Selector/5 -> [steigung]  "<steigung>"
  [i_getriebe] -> Bus Creator/2  "i_getriebe"
  [fps] -> Bus Creator/3  "fps"
  [v] -> Bus Creator/4  "v"
  [steigung] -> Bus Creator/5  "steigung"
  Bus Creator/1 -> OUT/1
  Bus Selector/6 -> [position_runde]  "<position_runde>"
  [position_runde] -> Bus Creator/6  "position_runde"
  Bus Selector/7 -> [radius]  "<radius>"
  [radius] -> Bus Creator/7  "radius"
  Bus Selector/8 -> [hoehenradius]  "<hoehenradius>"
  [hoehenradius] -> Bus Creator/8  "hoehenradius"

== system Model2_V032_R_T4/Fahr-Dynamik/Widerstände über Ausrollkurven ==
  note: Fahrwiderstände
  In1 : Inport
  Bus Selector : BusSelector  OutputSignals=v
  Constant14 : Constant  Value=ausrollen_a_v
  MATLAB Function : MATLAB Function  TreatAsAtomicUnit=on
  Out1 : Outport  VectorParamsAs1DForOutWhenUnconnected=off
  tag scope: F_W_ausrollkurven=global
  wires:
  In1/1 -> Bus Selector/1
  Bus Selector/1 -> [v]  "<v>"
  MATLAB Function/1(F_W_ausrollkurven) -> [F_W_ausrollkurven]
  [F_W_ausrollkurven] -> Out1/1
  [v] -> MATLAB Function/1(v)
  Constant14/1 -> MATLAB Function/2(ausrollen_a_v)

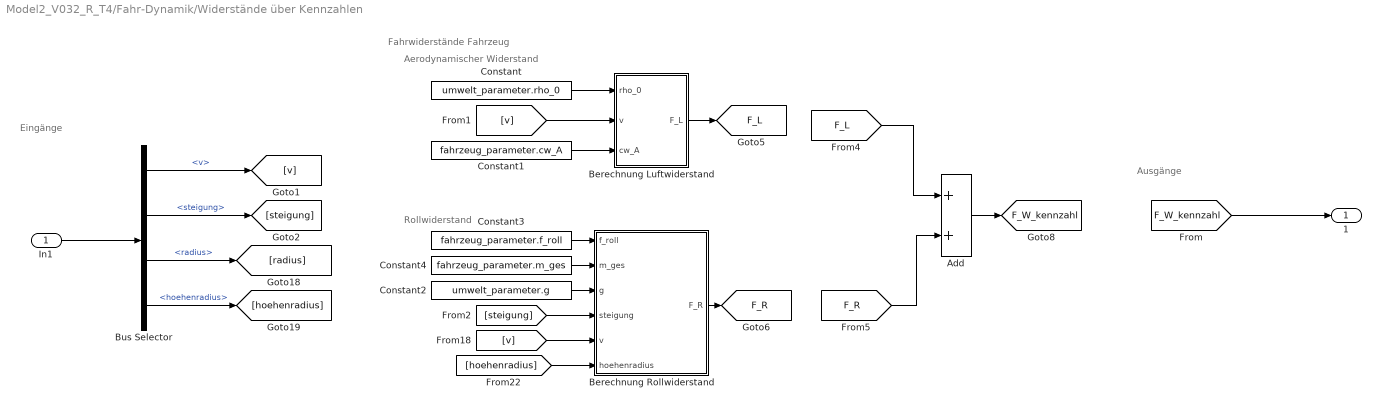
== system Model2_V032_R_T4/Fahr-Dynamik/Widerstände über Kennzahlen ==
  note: Aerodynamischer Widerstand
  note: Rollwiderstand
  note: Fahrwiderstände Fahrzeug
  note: Eingänge
  note: Ausgänge
  In1 : Inport
  Add : Sum
  Berechnung Luftwiderstand : MATLAB Function  TreatAsAtomicUnit=on
  Berechnung Rollwiderstand : MATLAB Function  TreatAsAtomicUnit=on
  Bus Selector : BusSelector  OutputSignals=v,steigung,radius,hoehenradius
  Constant : Constant  Value=umwelt_parameter.rho_0
  Constant1 : Constant  Value=fahrzeug_parameter.cw_A
  Constant2 : Constant  Value=umwelt_parameter.g
  Constant3 : Constant  Value=fahrzeug_parameter.f_roll
  Constant4 : Constant  Value=fahrzeug_parameter.m_ges
  1 : Outport  VectorParamsAs1DForOutWhenUnconnected=off
  tag scope: F_L=global, F_R=global, F_W_kennzahl=global
  wires:
  [hoehenradius] -> Berechnung Rollwiderstand/6(hoehenradius)
  Constant3/1 -> Berechnung Rollwiderstand/1(f_roll)
  [F_L] -> Add/1
  Constant4/1 -> Berechnung Rollwiderstand/2(m_ges)
  Constant1/1 -> Berechnung Luftwiderstand/3(cw_A)
  Constant/1 -> Berechnung Luftwiderstand/1(rho_0)
  Constant2/1 -> Berechnung Rollwiderstand/3(g)
  Berechnung Rollwiderstand/1(F_R) -> [F_R]
  Add/1 -> [F_W_kennzahl]
  [v] -> Berechnung Rollwiderstand/5(v)
  Berechnung Luftwiderstand/1(F_L) -> [F_L]
  [steigung] -> Berechnung Rollwiderstand/4(steigung)
  [F_R] -> Add/2
  [v] -> Berechnung Luftwiderstand/2(v)
  Bus Selector/4 -> [hoehenradius]  "<hoehenradius>"
  Bus Selector/2 -> [steigung]  "<steigung>"
  Bus Selector/3 -> [radius]  "<radius>"
  Bus Selector/1 -> [v]  "<v>"
  In1/1 -> Bus Selector/1
  [F_W_kennzahl] -> 1/1

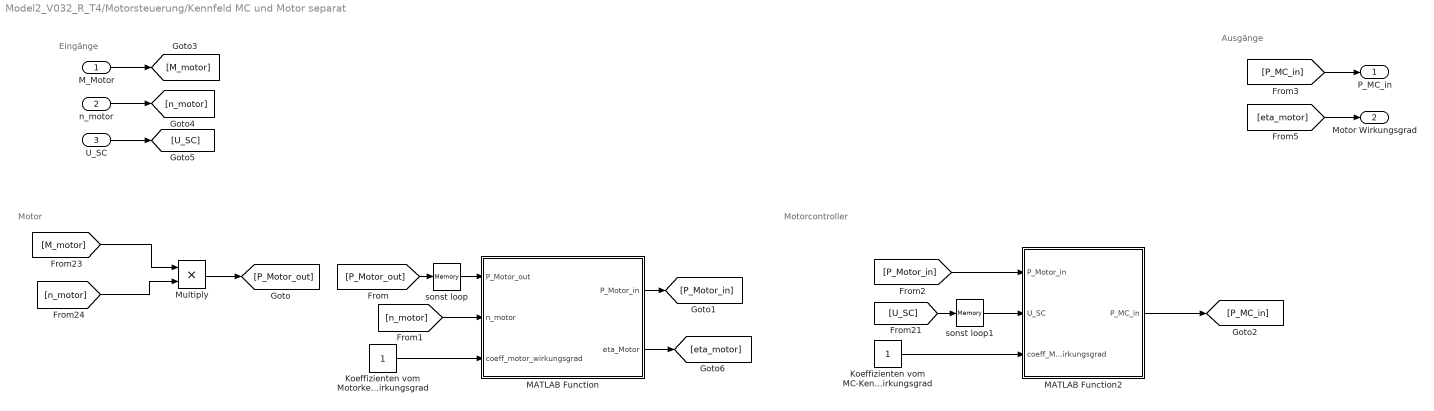
== system Model2_V032_R_T4/Motorsteuerung/Kennfeld MC und Motor separat ==
  note: Motor
  note: Motorcontroller
  note: Eingänge
  note: Ausgänge
  M_Motor : Inport
  n_motor : Inport  Port=2
  U_SC : Inport  Port=3
  Koeffizienten vom MC-Kennfeld Wirkungsgrad : Constant
  Koeffizienten vom Motorkennfeld Wirkungsgrad : Constant
  MATLAB Function : MATLAB Function  TreatAsAtomicUnit=on
  MATLAB Function2 : MATLAB Function  TreatAsAtomicUnit=on
  Multiply : Product
  sonst loop : Memory
  sonst loop1 : Memory
  P_MC_in : Outport  VectorParamsAs1DForOutWhenUnconnected=off
  Motor Wirkungsgrad : Outport  Port=2  VectorParamsAs1DForOutWhenUnconnected=off
  wires:
  [M_motor] -> Multiply/1
  [n_motor] -> Multiply/2
  Multiply/1 -> [P_Motor_out]
  [P_Motor_out] -> sonst loop/1
  [n_motor] -> MATLAB Function/2(n_motor)
  Koeffizienten vom Motorkennfeld Wirkungsgrad/1 -> MATLAB Function/3(coeff_motor_wirkungsgrad)
  MATLAB Function/1(P_Motor_in) -> [P_Motor_in]
  [P_Motor_in] -> MATLAB Function2/1(P_Motor_in)
  [U_SC] -> sonst loop1/1
  Koeffizienten vom MC-Kennfeld Wirkungsgrad/1 -> MATLAB Function2/3(coeff_MC_wirkungsgrad)
  MATLAB Function2/1(P_MC_in) -> [P_MC_in]
  M_Motor/1 -> [M_motor]
  n_motor/1 -> [n_motor]
  U_SC/1 -> [U_SC]
  [P_MC_in] -> P_MC_in/1
  [eta_motor] -> Motor Wirkungsgrad/1
  MATLAB Function/2(eta_Motor) -> [eta_motor]
  sonst loop/1 -> MATLAB Function/1(P_Motor_out)
  sonst loop1/1 -> MATLAB Function2/2(U_SC)

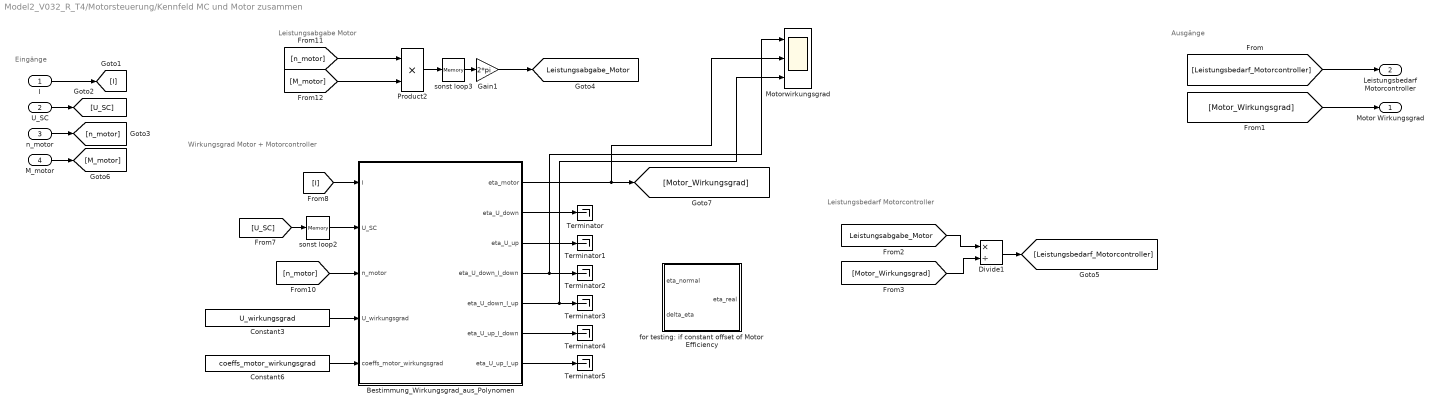
== system Model2_V032_R_T4/Motorsteuerung/Kennfeld MC und Motor zusammen ==
  note: Eingänge
  note: Ausgänge
  note: Leistungsabgabe Motor
  note: Leistungsbedarf Motorcontroller
  note: Wirkungsgrad Motor + Motorcontroller
  I : Inport
  U_SC : Inport  Port=2
  n_motor : Inport  Port=3
  M_motor : Inport  Port=4
  Bestimmung_Wirkungsgrad_aus_Polynomen : MATLAB Function  TreatAsAtomicUnit=on
  Constant3 : Constant  Value=U_wirkungsgrad  VectorParams1D=off
  Constant6 : Constant  Value=coeffs_motor_wirkungsgrad  VectorParams1D=off
  Divide1 : Product  Inputs=*/
  Gain1 : Gain  Gain=2*pi
  Motorwirkungsgrad : Scope  NumInputPorts=3
  Product2 : Product
  Terminator{,1..5} (6 alike) : Terminator
  for testing: if constant offset of Motor Efficiency : MATLAB Function  TreatAsAtomicUnit=on
  sonst loop2 : Memory
  sonst loop3 : Memory
  Motor Wirkungsgrad : Outport  VectorParamsAs1DForOutWhenUnconnected=off
  Leistungsbedarf Motorcontroller : Outport  Port=2  VectorParamsAs1DForOutWhenUnconnected=off
  tag scope: Leistungsabgabe_Motor=global
  wires:
  I/1 -> [I]
  U_SC/1 -> [U_SC]
  n_motor/1 -> [n_motor]
  [Leistungsbedarf_Motorcontroller] -> Leistungsbedarf Motorcontroller/1
  [Motor_Wirkungsgrad] -> Motor Wirkungsgrad/1
  M_motor/1 -> [M_motor]
  [U_SC] -> sonst loop2/1
  sonst loop2/1 -> Bestimmung_Wirkungsgrad_aus_Polynomen/2(U_SC)
  [I] -> Bestimmung_Wirkungsgrad_aus_Polynomen/1(I)
  [n_motor] -> Bestimmung_Wirkungsgrad_aus_Polynomen/3(n_motor)
  Constant3/1 -> Bestimmung_Wirkungsgrad_aus_Polynomen/4(U_wirkungsgrad)
  Constant6/1 -> Bestimmung_Wirkungsgrad_aus_Polynomen/5(coeffs_motor_wirkungsgrad)
  Bestimmung_Wirkungsgrad_aus_Polynomen/2(eta_U_down) -> Terminator/1
  Bestimmung_Wirkungsgrad_aus_Polynomen/3(eta_U_up) -> Terminator1/1
  Bestimmung_Wirkungsgrad_aus_Polynomen/4(eta_U_down_I_down) -> Motorwirkungsgrad/1, Terminator2/1
  Bestimmung_Wirkungsgrad_aus_Polynomen/5(eta_U_down_I_up) -> Motorwirkungsgrad/3, Terminator3/1
  Bestimmung_Wirkungsgrad_aus_Polynomen/6(eta_U_up_I_down) -> Terminator4/1
  Bestimmung_Wirkungsgrad_aus_Polynomen/7(eta_U_up_I_up) -> Terminator5/1
  Bestimmung_Wirkungsgrad_aus_Polynomen/1(eta_motor) -> Motorwirkungsgrad/2, [Motor_Wirkungsgrad]
  sonst loop3/1 -> Gain1/1
  [M_motor] -> Product2/2
  [n_motor] -> Product2/1
  Product2/1 -> sonst loop3/1
  Gain1/1 -> [Leistungsabgabe_Motor]
  Divide1/1 -> [Leistungsbedarf_Motorcontroller]
  [Leistungsabgabe_Motor] -> Divide1/1
  [Motor_Wirkungsgrad] -> Divide1/2

== matlab function Model2_V032_R_T4/Fahrer // Strategie/Zwangsgas berücksichtigen ==
  data: fps_neu input; fps_alt input; fps output; fertige_runden input; wegpunkt input; zwangsgas input; anzahl_runden_gesamt input; tstartstop output; v input; v_alt input; v_durch input; clock input; t_stop_start_alt input; ignore_zwangsausrollen output; zwangsgas_i output; ignore_zwangsausrollen_alt input
function [fps, tstartstop, ignore_zwangsausrollen, zwangsgas_i] = fcn( fps_neu , fps_alt, fertige_runden , wegpunkt , zwangsgas , anzahl_runden_gesamt, v, v_alt, v_durch, clock, t_stop_start_alt,ignore_zwangsausrollen_alt )
%% Zwangsgas berücksichtigen
% Hydro2Motion
% Prototyp: Homer
% Stand: 23.01.2020
% edited: Robin Nedella

%% Eingang
% fps_neu:                  [-]     in der Strategie vorgegebene fps (0: kein Gas, 1: Gas)
% fertige_runden:           [-]     Anzahl der bereits absolvierten Runden
% wegpunkt:                 [-]     Zeilennummer des letzten Wegpunktes aus dem strecke-Struct, welcher zuletzt passiert wurde
% zwangsgas:                [-]     Zwangsgas-Matrix
% anzahl_runden_gesamt:     [-]     Gesamtzahl der Runden

%% Ausgang
% fps:                      [-]     kommandierte Fahrpedalstellung

%% Berechnung
% Zwangsgas hat Vorrang
fps = fps_neu;  % Initialisierung

% Abfrage, ob Simulation fertig ist
if fertige_runden == anzahl_runden_gesamt
    fps = 0;
elseif zwangsgas(wegpunkt , fertige_runden + 1) == 1
    % Zwangsgas überschreibt fps, wenn Zwangsgas zum aktuellen Wegpunkt in der aktuellen Runde 1 ist
    fps = 1;
elseif zwangsgas(wegpunkt , fertige_runden + 1) == 2
    % ZwangsAUSROLLEN!!!
    fps = 0;
end

% Datenspeicherung für Simulationsauswertung
if fertige_runden < anzahl_runden_gesamt
    zwangsgas_i = zwangsgas(wegpunkt , fertige_runden + 1);
else
    zwangsgas_i = 0;
end

%% Bremsen und Stehen bleiben
tstartstop = clock;    
% 15 Sekunden stehen bleiben
stopdelay = 15;
ignore_zwangsausrollen = 0;

if v <= 0
    if  v_alt > 0
        % Stehenbleiben erkannt
        tstartstop = t_stop_start_alt;
        ignore_zwangsausrollen = 1;
        disp("Stehen geblieben");
    end
elseif ignore_zwangsausrollen_alt == 1
    % nach stopdelay sec.
    % Während Beschleunigen wegen Stehenbleiben, aber noch nicht bei v_durch
    % if ((clock - tstartstop) >= stopdelay)  && v < v_durch
    if v < (v_durch)
        ignore_zwangsausrollen = 1;
        fps = 1;
    else
        ignore_zwangsausrollen = 0; % weiter egal
    end
else
%     % Prüfen ob gewollte Standzeit erreicht wird und dann wieder Gasgeben
%     % bis v_durch
%     tstartstop = t_stop_start_alt;
%     if ((clock - tstartstop) >= stopdelay) && v <= v_durch
%         fps = 1;
%         ignore_zwangsausrollen = 1;
%     end
end

end

== matlab function Model2_V032_R_T4/Fahrer // Strategie/Zwangsgas berücksichtigen1 ==
  data: fps_neu input; fps output; fertige_runden input; wegpunkt input; zwangsgas input; anzahl_runden_gesamt input
function fps  = fcn( fps_neu , fertige_runden , wegpunkt , zwangsgas , anzahl_runden_gesamt )
%% Zwangsgas berücksichtigen
% Hydro2Motion
% Prototyp: Homer
% Stand: 23.01.2020
% edited: Robin Nedella

%% Eingang
% fps_neu:                  [-]     in der Strategie vorgegebene fps (0: kein Gas, 1: Gas)
% fertige_runden:           [-]     Anzahl der bereits absolvierten Runden
% wegpunkt:                 [-]     Zeilennummer des letzten Wegpunktes aus dem strecke-Struct, welcher zuletzt passiert wurde
% zwangsgas:                [-]     Zwangsgas-Matrix
% anzahl_runden_gesamt:     [-]     Gesamtzahl der Runden

%% Ausgang
% fps:                      [-]     kommandierte Fahrpedalstellung

%% Berechnung
% Zwangsgas hat Vorrang
    fps = fps_neu;  % Initialisierung
    
    % Abfrage, ob Simulation fertig ist
    if fertige_runden == anzahl_runden_gesamt
        fps = 0;
    elseif zwangsgas(wegpunkt , fertige_runden + 1) == 1
        % Zwangsgas überschreibt fps, wenn Zwangsgas zum aktuellen Wegpunkt in der aktuellen Runde 1 ist
        fps = 1;
    elseif zwangsgas(wegpunkt , fertige_runden + 1) == 2
        % ZwangsAUSROLLEN!!!
        fps = 0;
    end
    
end
